simulink model "SRS_simulation"  (R2019a)
settings: Solver=VariableStepAuto  StartTime=0.0  StopTime=180  RelTol=1e-3
libraries: dsparch4 x2, simulink x1
settings Model: Creator=patri  LastModifiedBy=patri

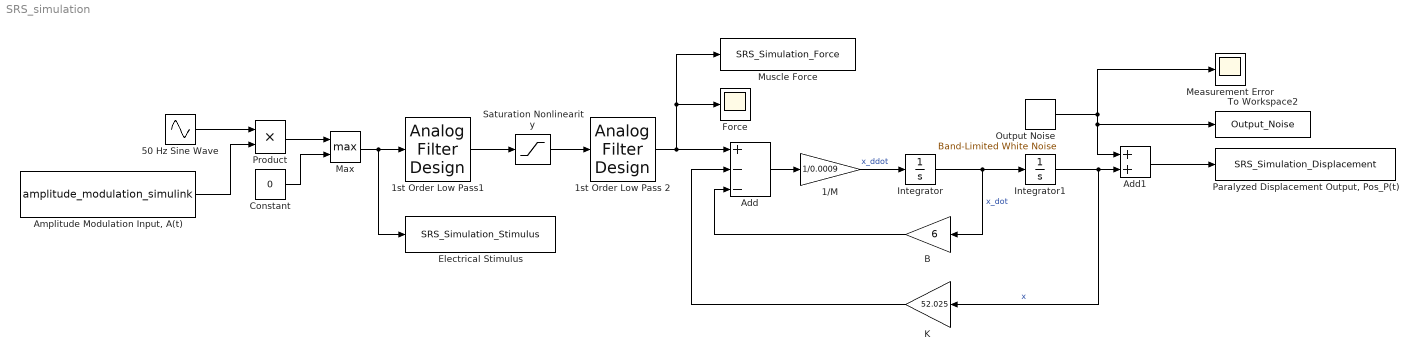
== system SRS_simulation ==
  1/M : Gain  Gain=1/0.0009
  1st Order Low Pass 2 : dsparch4/Analog Filter Design  method=Butterworth  filttype=Lowpass  N=1  Wlo=6.28*4  Whi=80  Rp=2  Rs=40
  1st Order Low Pass1 : dsparch4/Analog Filter Design  method=Butterworth  filttype=Lowpass  N=1  Wlo=6.28*4  Whi=80  Rp=2  Rs=40
  50 Hz Sine Wave : Sin  Frequency=314.16  SampleTime=0.001
  Add : Sum  Inputs=+--
  Add1 : Sum
  "Amplitude Modulation Input, A(t)" : FromWorkspace  VariableName=amplitude_modulation_simulink  SampleTime=0.001
  B : Gain  Gain=6
  Constant : Constant  Value=0
  Electrical Stimulus : ToWorkspace  VariableName=SRS_Simulation_Stimulus  SampleTime=0.001
  Force : Scope
  Integrator : Integrator
  Integrator1 : Integrator
  "K                " : Gain  Gain=52.025
  Max : MinMax  Function=max  Inputs=2
  Measurement Error : Scope
  Muscle Force : ToWorkspace  VariableName=SRS_Simulation_Force  SampleTime=0.001
  Output Noise : simulink/Sources/Band-Limited White Noise  Cov=set_output_noise_power  Ts=0.001  seed=223341
  "Paralyzed Displacement Output, Pos_P(t)" : ToWorkspace  VariableName=SRS_Simulation_Displacement  SampleTime=0.001
  Product : Product
  Saturation Nonlinearity : Saturate  UpperLimit=0.52  LowerLimit=0
  To Workspace2 : ToWorkspace  VariableName=Output_Noise  SampleTime=0.001
  wires:
  Saturation Nonlinearity/1 -> 1st Order Low Pass 2/1
  1st Order Low Pass1/1 -> Saturation Nonlinearity/1
  Max/1 -> Electrical Stimulus/1, 1st Order Low Pass1/1
  1/M/1 -> Integrator/1  "x_ddot"
  Integrator/1 -> B/1, Integrator1/1  "x_dot"
  "K                "/1 -> Add/2
  Integrator1/1 -> "K                "/1, Add1/2  "x"
  Add/1 -> 1/M/1
  B/1 -> Add/3
  Add1/1 -> "Paralyzed Displacement Output, Pos_P(t)"/1
  Output Noise/1 -> To Workspace2/1, Add1/1, Measurement Error/1
  1st Order Low Pass 2/1 -> Add/1, Muscle Force/1, Force/1
  "Amplitude Modulation Input, A(t)"/1 -> Product/2
  50 Hz Sine Wave/1 -> Product/1
  Product/1 -> Max/1
  Constant/1 -> Max/2
